simulink model "OfflineEstimator"  (R2020a)
settings: Solver=ode1be  StartTime=0.0  StopTime=simParams.duration.Value  FixedStep=0.00005  MaxStep=0.0005*sqrt(simParams.lengthScaleFactor.Value)  RelTol=1e-3  AbsTol=1e-3
undefined symbols (not defined in the file or in its folder): bridlePosVec, CMposVec, env, experimentalDataIsInput, externalDataIsInput, initPosKite, initVelKite, las, LEposIMU, linThrNodeCorrVec, NNodeTether, NNodeTether_cl, numObsThrNodes, obsLASphidotInit, obsLASphiInit, obsLASthetadotInit, obsLASthetaInit, ObsLink1DFlowVec, OBSTETHER, Obsthr, tow_start_time
libraries: vrlib x5, lineAngleSensor x5, dspsrcs4 x4, sharedutil x3, nodeDragForce_ul x3, nodeNetBuoyForce_ul x3, nodePosToLinkPos_ul x3, nodeSpringDamperForce_ul x3, eeGeneralControl x3, stateEstimation x3, dspsigops x3, thrNodeMass_ul x2
(part 1 of 2)
settings Model: SimulationMode=accelerator  PauseTimes=15  PacingRate=1000  ExtModeTrigDuration=100  Creator=mcobb  LastModifiedBy=Zak
settings SolverCC: AlgebraicLoopSolver=LineSearch  SolverResetMethod=Robust
settings DataIOCC: SaveFormat=StructureWithTime  SaveOutput=off  DSMLogging=off  StateSaveName=tmp_raccel_xout
settings OptimizationCC: EfficientMapNaN2IntZero=off
settings DebuggingCC: SignalRangeChecking=error  AlgebraicLoopMsg=none  ArtificialAlgebraicLoopMsg=none  ArithmeticOperatorsInVariantConditions=warning
settings HardwareCC: TargetBitPerPointer=64  TargetBitPerSizeT=64  TargetBitPerPtrDiffT=64  TargetLongLongMode=on  TargetIntDivRoundTo=Zero  TargetEndianess=LittleEndian  TargetWordSize=64  TargetHWDeviceType=MATLAB Host  ProdEqTarget=off
settings SFSimCC: CustomCodeUndefinedFunction=UseInterfaceOnly
settings CodeAppCC: MaxIdLength=128
settings GRTTargetCC: CombineOutputUpdateFcns=off  GRTInterface=on

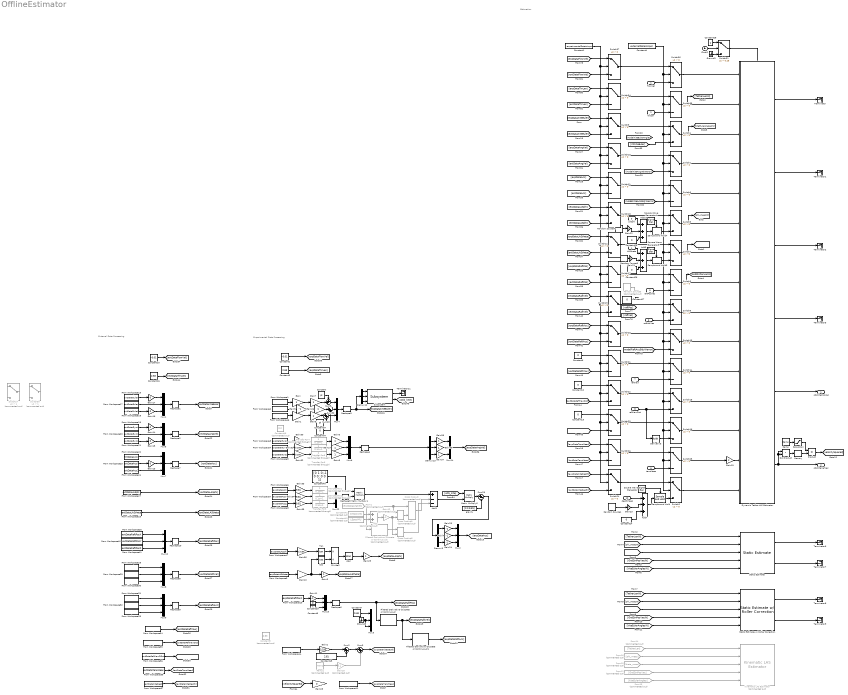
== system OfflineEstimator ==
  note: Estimation
  note: Experimental Data Processing
  note: External Data Processing
  flowVel : Inport
  thrLen : Inport  Port=2
  LASphi : Inport  Port=3
  LAStheta : Inport  Port=4
  raftPosVec : Inport  Port=5
  raftVelVec : Inport  Port=6
  raftYaw : Inport  Port=7
  raftYawDot : Inport  Port=8
  tensMeas : Inport  Port=9
  depthMeas : Inport  Port=10
  Add : Sum  Commented=on
  Add1 : Sum  Inputs=+--
  Add10 : Sum  Inputs=+++
  Add7 : Sum  Inputs=+++
  Add9 : Sum  Inputs=+++
  Atan : Trigonometry  Operator=atan
  Clock2 : Clock
  Constant : Constant  Value=pi
  Constant1 : Constant  Value=experimentalDataIsInput
  Constant10 : Constant  Value=-0.01
  Constant{6,12..13,24..27,29,47} (9 alike) : Constant  Value=0
  Constant16 : Constant  Value=2.63
  Constant2 : Constant  Value=-0.01
  Constant28 : Constant
  Constant3 : Constant  Value=2.63
  Constant37 : Constant  Value=pi
  Constant4 : Constant  Value=externalDataIsInput
  Constant40 : Constant  Value=[0 1 0;-1 0 0; 0 0 1]
  Constant42 : Constant  Commented=on  Value=CMposVec
  Constant43 : Constant  Commented=on  Value=LEposIMU
  Constant45 : Constant  Value=2.81
  Constant46 : Constant  Commented=on  Value=0.2
  Constant5 : Constant  Commented=on  Value=2.63
  Constant7 : Constant  Value=0.48
  Constant8 : Constant  Value=3
  Cos : Trigonometry  Operator=cos
  Cross Product : vrlib/Utilities/Cross Product  Commented=on
  Cross Product1 : vrlib/Utilities/Cross Product  Commented=on
  Cross Product2 : vrlib/Utilities/Cross Product  Commented=on
  Demux12 : Demux  Outputs=3
  Demux13 : Demux  Outputs=3
  Demux3 : Demux  Outputs=3
  Derivative : Derivative
  Divide2 : Product  Inputs=*/
  Dot Product : DotProduct  InputSameDT=on  OutDataTypeStr=Inherit: Inherit via internal rule
  Dynamic Tether LAS Estimator : Subsystem  AncestorBlock=lineAngleSensorObserver/lineAngleSensorObserver  mask{las=las, env=env}
      mask prompts: las "LAS Object"; env "Environment"
  Filtered Derivative (Discrete or Continuous) : eeGeneralControl/Filtered Derivative (Discrete or Continuous)  K=1  T=0.5  B=inf  A=-inf  minRatio=10  init_option=Inherited from block input  x0=0  Ts=-1
      settings: SourceProductBaseCode=PS
  Filtered Derivative (Discrete or Continuous)1 : eeGeneralControl/Filtered Derivative (Discrete or Continuous)  K=1  T=0.5  B=inf  A=-inf  minRatio=10  init_option=Inherited from block input  x0=0  Ts=-1
      settings: SourceProductBaseCode=PS
  Filtered Derivative (Discrete or Continuous)2 : eeGeneralControl/Filtered Derivative (Discrete or Continuous)  Commented=on  K=1  T=0.5  B=inf  A=-inf  minRatio=10  init_option=Inherited from block input  x0=0  Ts=-1
      settings: SourceProductBaseCode=PS
  From Workspace1 : FromWorkspace  VariableName=expDataEulerX  SampleTime=0.001  Interpolate=off  ZeroCross=off  OutputAfterFinalValue=Holding final value
  From Workspace10 : FromWorkspace  VariableName=expDataRaftPosX  SampleTime=0.001  Interpolate=off  ZeroCross=off  OutputAfterFinalValue=Holding final value
  From Workspace11 : FromWorkspace  VariableName=expDataTensMeas  SampleTime=0.001  Interpolate=off  ZeroCross=off  OutputAfterFinalValue=Holding final value
  From Workspace14 : FromWorkspace  VariableName=expDataKiteDepth  SampleTime=0.001  Interpolate=off  ZeroCross=off  OutputAfterFinalValue=Holding final value
  From Workspace15 : FromWorkspace  VariableName=extDataEulerX  SampleTime=0.001  Interpolate=off  ZeroCross=off  OutputAfterFinalValue=Holding final value
  From Workspace17 : FromWorkspace  VariableName=extDataEulerY  SampleTime=0.001  Interpolate=off  ZeroCross=off  OutputAfterFinalValue=Holding final value
  From Workspace18 : FromWorkspace  VariableName=extDataEulerZ  SampleTime=0.001  Interpolate=off  ZeroCross=off  OutputAfterFinalValue=Holding final value
  From Workspace19 : FromWorkspace  VariableName=extDataGyroX  SampleTime=0.001  Interpolate=off  ZeroCross=off  OutputAfterFinalValue=Holding final value
  From Workspace2 : FromWorkspace  VariableName=expDataEulerY  SampleTime=0.001  Interpolate=off  ZeroCross=off  OutputAfterFinalValue=Holding final value
  From Workspace20 : FromWorkspace  VariableName=extDataGyroY  SampleTime=0.001  Interpolate=off  ZeroCross=off  OutputAfterFinalValue=Holding final value
  From Workspace21 : FromWorkspace  VariableName=extDataGyroZ  SampleTime=0.001  Interpolate=off  ZeroCross=off  OutputAfterFinalValue=Holding final value
  From Workspace22 : FromWorkspace  VariableName=extDataAccX  SampleTime=0.001  Interpolate=off  ZeroCross=off  OutputAfterFinalValue=Holding final value
  From Workspace23 : FromWorkspace  VariableName=extDataAccY  SampleTime=0.001  Interpolate=off  ZeroCross=off  OutputAfterFinalValue=Holding final value
  From Workspace24 : FromWorkspace  VariableName=extDataAccZ  SampleTime=0.001  Interpolate=off  ZeroCross=off  OutputAfterFinalValue=Holding final value
  From Workspace25 : FromWorkspace  VariableName=extDataLAStheta  SampleTime=0.001  Interpolate=off  ZeroCross=off  OutputAfterFinalValue=Holding final value
  From Workspace26 : FromWorkspace  VariableName=extDataRaftPosX  SampleTime=0.001  Interpolate=off  ZeroCross=off  OutputAfterFinalValue=Holding final value
  From Workspace27 : FromWorkspace  VariableName=extDataLASphi  SampleTime=0.001  Interpolate=off  ZeroCross=off  OutputAfterFinalValue=Holding final value
  From Workspace28 : FromWorkspace  VariableName=extDataRaftVelX  SampleTime=0.001  Interpolate=off  ZeroCross=off  OutputAfterFinalValue=Holding final value
  From Workspace29 : FromWorkspace  VariableName=extDataRaftVelY  SampleTime=0.001  Interpolate=off  ZeroCross=off  OutputAfterFinalValue=Holding final value
  From Workspace3 : FromWorkspace  VariableName=expDataGyroX  SampleTime=0.001  Interpolate=off  ZeroCross=off  OutputAfterFinalValue=Holding final value
  From Workspace30 : FromWorkspace  VariableName=extDataRaftVelZ  SampleTime=0.001  Interpolate=off  ZeroCross=off  OutputAfterFinalValue=Holding final value
  From Workspace31 : FromWorkspace  VariableName=extDataRaftAccX  SampleTime=0.001  Interpolate=off  ZeroCross=off  OutputAfterFinalValue=Holding final value
  From Workspace32 : FromWorkspace  VariableName=extDataRaftAccY  SampleTime=0.001  Interpolate=off  ZeroCross=off  OutputAfterFinalValue=Holding final value
  From Workspace33 : FromWorkspace  VariableName=extDataRaftAccZ  SampleTime=0.001  Interpolate=off  ZeroCross=off  OutputAfterFinalValue=Holding final value
  From Workspace34 : FromWorkspace  VariableName=extDataRaftYaw  SampleTime=0.001  Interpolate=off  ZeroCross=off  OutputAfterFinalValue=Holding final value
  From Workspace35 : FromWorkspace  VariableName=extDataRaftYawDot  SampleTime=0.001  Interpolate=off  ZeroCross=off  OutputAfterFinalValue=Holding final value
  From Workspace36 : FromWorkspace  VariableName=extDataRaftYawDDot  SampleTime=0.001  Interpolate=off  ZeroCross=off  OutputAfterFinalValue=Holding final value
  From Workspace37 : FromWorkspace  VariableName=extDataKiteDepth  SampleTime=0.001  Interpolate=off  ZeroCross=off  OutputAfterFinalValue=Holding final value
  From Workspace39 : FromWorkspace  VariableName=extDataTensMeas  SampleTime=0.001  Interpolate=off  ZeroCross=off  OutputAfterFinalValue=Holding final value
  From Workspace4 : FromWorkspace  VariableName=expDataGyroY  SampleTime=0.001  Interpolate=off  ZeroCross=off  OutputAfterFinalValue=Holding final value
  From Workspace40 : FromWorkspace  VariableName=extDataRaftPosY  SampleTime=0.001  Interpolate=off  ZeroCross=off  OutputAfterFinalValue=Holding final value
  From Workspace41 : FromWorkspace  VariableName=extDataRaftPosZ  SampleTime=0.001  Interpolate=off  ZeroCross=off  OutputAfterFinalValue=Holding final value
  From Workspace46 : FromWorkspace  VariableName=expDataEulerZ  SampleTime=0.001  Interpolate=off  ZeroCross=off  OutputAfterFinalValue=Holding final value
  From Workspace47 : FromWorkspace  VariableName=expDataLASphi  SampleTime=0.001  Interpolate=off  ZeroCross=off  OutputAfterFinalValue=Holding final value
  From Workspace5 : FromWorkspace  VariableName=expDataGyroZ  SampleTime=0.001  Interpolate=off  ZeroCross=off  OutputAfterFinalValue=Holding final value
  From Workspace6 : FromWorkspace  VariableName=expDataAccX  SampleTime=0.001  Interpolate=off  ZeroCross=off  OutputAfterFinalValue=Holding final value
  From Workspace7 : FromWorkspace  VariableName=expDataAccY  SampleTime=0.001  Interpolate=off  ZeroCross=off  OutputAfterFinalValue=Holding final value
  From Workspace8 : FromWorkspace  VariableName=expDataAccZ  SampleTime=0.001  Interpolate=off  ZeroCross=off  OutputAfterFinalValue=Holding final value
  From Workspace9 : FromWorkspace  VariableName=expDataLAStheta  SampleTime=0.001  Interpolate=off  ZeroCross=off  OutputAfterFinalValue=Holding final value
  From1 : From  Commented=on  GotoTag=expDataAngVel
  From12 : From  Commented=on  GotoTag=GndStnPosVec
  From13 : From  Commented=on  GotoTag=kiteEulerAngles
  From14 : From  Commented=on  GotoTag=TetherLen
  From15 : From  Commented=on  GotoTag=theta_meas
  From16 : From  Commented=on  GotoTag=phi_meas
  Gain{,3,5..8,26..27,29,37..39} (12 alike) : Gain
  Gain1 : Gain  Gain=-pi/180
  Gain10 : Gain  Gain=-pi/180
  Gain{4,9,11,24..25} (5 alike) : Gain  Gain=-1
  Gain12 : Gain  Commented=on  Gain=-1
  Gain{13..17,21..23,28} (9 alike) : Gain  Gain=0
  Gain18 : Gain  Commented=on  Gain=0.1
  Gain19 : Gain  Gain=2
  Gain2 : Gain  Gain=-1/100
  Gain{30..32,36} (4 alike) : Gain  Gain=pi/180
  Gain33 : Gain  Gain=9.81
  Gain34 : Gain  Gain=9.81
  Gain35 : Gain  Gain=9.81
  Ground3 : Ground
  Ground8 : Ground
  Kinematic LAS Estimator : stateEstimation/State Estimation/Kinematic LAS Estimator  Commented=on  SystemSampleTime=-1  Latency=0  AutoFrameSizeCalculation=off
  Matrix Multiply1 : Product  Multiplication=Matrix(*)
  Matrix Multiply6 : Product  Multiplication=Matrix(*)
  Memory : Memory
  Mux{1..10,22..24} (13 alike) : Mux  Inputs=3
  Product : Product
  Ramp : simulink/Sources/Ramp  slope=0.1  start=0  InitialOutput=0
  Ramp1 : simulink/Sources/Ramp  Commented=on  slope=0.5  start=10  InitialOutput=0
  Random Source1 : dspsrcs4/Random Source  SrcType=Gaussian  NormMethod=Ziggurat  CltLength=12  MinVal=0  MaxVal=1  MeanVal=0  VarVal=1e-6  RepMode=Not repeatable  rawSeed=1  IsInherit=off  SampMode=Continuous  SampTime=0.01  SampFrame=1  DataType=Double  OutComplex=Real  OutputFrames=off
  Random Source3 : dspsrcs4/Random Source  SrcType=Gaussian  NormMethod=Ziggurat  CltLength=12  MinVal=0  MaxVal=1  MeanVal=0  VarVal=(0.01*3.14/180)^2  RepMode=Not repeatable  rawSeed=1  IsInherit=off  SampMode=Continuous  SampTime=0.01  SampFrame=1  DataType=Double  OutComplex=Real  OutputFrames=off
  Random Source4 : dspsrcs4/Random Source  SrcType=Gaussian  NormMethod=Ziggurat  CltLength=12  MinVal=0  MaxVal=1  MeanVal=0  VarVal=(0.01*3.14/180)^2  RepMode=Not repeatable  rawSeed=1  IsInherit=off  SampMode=Continuous  SampTime=0.01  SampFrame=1  DataType=Double  OutComplex=Real  OutputFrames=off
  Random Source5 : dspsrcs4/Random Source  Commented=on  SrcType=Gaussian  NormMethod=Ziggurat  CltLength=12  MinVal=0  MaxVal=1  MeanVal=0  VarVal=1e-6  RepMode=Not repeatable  rawSeed=1  IsInherit=off  SampMode=Continuous  SampTime=0.01  SampFrame=1  DataType=Double  OutComplex=Real  OutputFrames=off
  Reshape{1..10} (10 alike) : Reshape  OutputDimensionality=Column vector (2-D)
  Sample and Hold : dspsigops/Sample and Hold  trig=Rising edge  initCond=0  latchinput=off
  Sample and Hold3 : dspsigops/Sample and Hold  trig=Rising edge  initCond=0  latchinput=off
  Sample and Hold4 : dspsigops/Sample and Hold  trig=Rising edge  initCond=0  latchinput=off
  Saturation : Saturate  UpperLimit=1  LowerLimit=0
  Square Wave Generator : SignalGenerator  WaveForm=square  Frequency=25
  Square Wave Generator3 : SignalGenerator  WaveForm=square  Frequency=25
  Square Wave Generator4 : SignalGenerator  WaveForm=square  Frequency=25
  Static Estimate : stateEstimation/State Estimation/Static Estimate  SystemSampleTime=-1  Latency=0  AutoFrameSizeCalculation=off
  Static Estimate w/ Roller Correction : stateEstimation/State Estimation/Static Estimate w// Roller Correction  SystemSampleTime=-1  Latency=0  AutoFrameSizeCalculation=off
  Subsystem : lineAngleSensorObserver/lineAngleSensorObserver/Subsystem  SystemSampleTime=-1  Latency=0  AutoFrameSizeCalculation=off
  Sum{2..3,28,30} (4 alike) : Sum  Inputs=|++
  Sum29 : Sum  Inputs=|+-
  Sum5 : Sum  Inputs=++|
  Switch{1..26,34..37} (30 alike) : Switch  Criteria=u2 > Threshold
  Switch27 : Switch  Commented=on  Criteria=u2 > Threshold  Threshold=1
  Switch30 : Switch  Commented=on  Criteria=u2 > Threshold  Threshold=1
  Switch31 : Switch  Criteria=u2 > Threshold  Threshold=0.25
  Tan : Trigonometry  Operator=tan
  Terminator{,1..3,6..9,11} (9 alike) : Terminator
  Transfer Fcn{1..6} (6 alike) : TransferFcn  Commented=through  Denominator=[0.1 1]
  gravity : Constant  Value=[0 0 9.81]
  obsKitePosVec : Outport
  obsKiteVelVec : Outport  Port=2
  wires:
  raftYaw/1 -> Switch14/3
  Switch3/1 -> [GndStnPosVecIN], Dynamic Tether LAS Estimator/8(raftPos)  "obsIN_RaftPos"
  Switch35/1 -> Dynamic Tether LAS Estimator/2(thrLen), [TetherLenIN]  "obsIN_obsThrLen"
  Constant4/1 -> Switch36/2, Switch35/2, Switch1/2, Switch6/2, Switch5/2, Switch7/2, Switch3/2, Switch13/2, Switch14/2, Switch15/2, Switch25/2, Switch2/2, Switch16/2, Switch8/2, Switch4/2
  Dynamic Tether LAS Estimator/2(phiDot) -> Terminator1/1  "obsOUT_LASphiDot"
  Dynamic Tether LAS Estimator/5(estKitePos) -> obsKitePosVec/1  "obsOUT_kitePosVec"
  Derivative/1 -> Switch16/3
  [extDataRaftYaw] -> Switch21/3
  Switch6/1 -> Dynamic Tether LAS Estimator/5(KiteAcc)  "obsIN_kiteAcc"
  Switch26/1 -> Switch25/1
  From Workspace41/1 -> Mux10/3
  From Workspace34/1 -> [extDataRaftYaw]
  Switch1/1 -> Dynamic Tether LAS Estimator/4(kiteAngVel)  "obsIN_kiteAngVel"
  Switch21/1 -> Switch14/1
  Constant6/1 -> Switch21/1
  Static Estimate w/ Roller Correction/1 -> Terminator8/1  "staticEstRollerOut_kitePosVec"
  Switch19/1 -> Switch8/1
  From Workspace29/1 -> Mux8/2
  From Workspace18/1 -> Gain16/1
  From Workspace17/1 -> Mux1/2
  Reshape10/1 -> [extDataRaftPos]
  Mux7/1 -> Reshape7/1
  Switch24/1 -> Switch2/1
  Mux5/1 -> Reshape2/1
  [expDataKiteEuler] -> Switch9/1
  From13/1 -> Kinematic LAS Estimator/5
  From16/1 -> Kinematic LAS Estimator/2
  Static Estimate w/ Roller Correction/2 -> Terminator9/1  "staticEstRollerOut_kiteVelVec"
  From12/1 -> Kinematic LAS Estimator/4
  From Workspace37/1 -> [extDataKiteDepth]
  [kiteEulerAnglesIN] -> Static Estimate w/ Roller Correction/5
  [kiteEulerAnglesIN] -> Static Estimate/5  "staticEstIn_eulerAnglesKite"
  From Workspace25/1 -> [extDataLAStheta]
  [theta_measIN] -> Static Estimate w/ Roller Correction/3
  flowVel/1 -> Switch36/3  "obsIN_flowVel"
  Switch4/1 -> Dynamic Tether LAS Estimator/3(kiteEulerAngles), [kiteEulerAnglesIN]  "obsIN_KiteEulerAngles"
  From Workspace21/1 -> Gain15/1
  Switch37/1 -> Switch36/1
  [extDataFlowVel] -> Switch37/3
  Gain22/1 -> Add10/2
  From Workspace15/1 -> Gain17/1
  Gain23/1 -> Add7/2
  [expDataAcc] -> Switch11/1
  From Workspace33/1 -> Mux9/3
  From Workspace26/1 -> Mux10/1
  Switch2/1 -> Dynamic Tether LAS Estimator/15(depthMeas)  "obsIN_kiteDepth"
  Switch9/1 -> Switch4/1
  Constant12/1 -> Switch22/1
  [extDataKiteDepth] -> Switch24/3
  Switch8/1 -> Dynamic Tether LAS Estimator/9(raftVel)  "obsIN_RaftVel"
  From Workspace28/1 -> Mux8/1
  [expDataRaftVel] -> Switch19/1
  tensMeas/1 -> Switch25/3
  From Workspace40/1 -> Mux10/2
  Switch13/1 -> Dynamic Tether LAS Estimator/10(raftAcc)  "obsIN_RaftAcc"
  From14/1 -> Kinematic LAS Estimator/1
  Square Wave Generator4/1 -> Sample and Hold4/Trigger
  Switch23/1 -> Switch16/1
  From Workspace23/1 -> Gain13/1
  [expDataTensMeas] -> Switch26/1
  Clock2/1 -> Switch31/2
  [modelKiteAccBdyWerror] -> Switch6/3
  Sample and Hold4/1 -> Switch5/3
  LASphi/1 -> Add10/1
  Mux10/1 -> Reshape10/1
  Switch36/1 -> Dynamic Tether LAS Estimator/1(flowSpd)  "obsIN_flowVel"
  Add10/1 -> Sample and Hold4/1
  Mux8/1 -> Reshape8/1
  Sample and Hold/1 -> Switch2/3
  Sample and Hold3/1 -> Switch7/3
  Static Estimate/2 -> Terminator7/1  "staticEstOut_kiteVelVec"
  From Workspace19/1 -> Gain14/1
  Constant28/1 -> Switch31/1
  Switch18/1 -> Switch5/1
  Random Source4/1 -> Gain22/1
  Random Source3/1 -> Gain21/1
  Constant26/1 -> Add9/3
  From Workspace31/1 -> Mux9/1
  Ground3/1 -> Switch31/3
  Switch10/1 -> Switch1/1
  Constant25/1 -> Add10/3
  Switch17/1 -> Switch3/1
  Square Wave Generator/1 -> Sample and Hold/Trigger
  Dynamic Tether LAS Estimator/1(phi) -> Terminator/1  "obsOUT_LASphi"
  Reshape7/1 -> [extDataAcc]
  [extDataRaftYawDot] -> Switch22/3
  From15/1 -> Kinematic LAS Estimator/3
  [expDataThrLen] -> Switch34/1
  depthMeas/1 -> Add7/1
  Dynamic Tether LAS Estimator/3(theta) -> Terminator2/1  "obsOUT_LAStheta"
  From Workspace36/1 -> [extDataRaftYawDDot]
  Switch12/1 -> Switch7/1
  [phi_measIN] -> Static Estimate w/ Roller Correction/2
  [expDataLASphi] -> Switch18/1
  Switch14/1 -> Dynamic Tether LAS Estimator/11(raftPsi)  "obsIN_RaftYaw"
  Random Source1/1 -> Gain23/1
  From Workspace27/1 -> [extDataLASphi]
  [extDataTensMeas] -> Switch26/3
  Static Estimate/1 -> Terminator6/1  "staticEstOut_kitePosVec"
  Dynamic Tether LAS Estimator/6(estKiteVel) -> obsKiteVelVec/1, Dot Product/1, Dot Product/2  "obsOUT_kiteVelVec"
  [extDataThrLen] -> Switch34/3
  Switch20/1 -> Switch13/1
  Dynamic Tether LAS Estimator/4(thetaDot) -> Terminator3/1  "obsOUT_LASthetaDot"
  Switch16/1 -> Dynamic Tether LAS Estimator/13(raftPsiDDot)  "obsIN_RaftYawDDot"
  Reshape8/1 -> [extDataRaftVel]
  Reshape1/1 -> [extDataKiteEuler]
  From Workspace24/1 -> Mux7/3
  From Workspace20/1 -> Mux5/2
  Switch7/1 -> [theta_measIN], Dynamic Tether LAS Estimator/7(LASthetaMeas)  "obsIN_LASthetaMeas"
  From Workspace22/1 -> Mux7/1
  [extDataRaftAcc] -> Switch20/3
  Switch15/1 -> Dynamic Tether LAS Estimator/12(raftPsiDot)  "obsIN_RaftYawDot"
  Constant13/1 -> Switch23/1
  [GndStnPosVecIN] -> Static Estimate/4  "staticEstIn_raftPosVec"
  [expDataLAStheta] -> Switch12/1
  Constant10/1 -> [extDataFlowVel]
  Add7/1 -> Sample and Hold/1
  Add9/1 -> Sample and Hold3/1
  [extDataRaftVel] -> Switch19/3
  From Workspace35/1 -> [extDataRaftYawDot]
  [extDataKiteEuler] -> Switch9/3
  raftVelVec/1 -> Switch8/3
  [TetherLenIN] -> Static Estimate/1  "staticEstIn_thrLen"
  LAStheta/1 -> Add9/1
  [extDataRaftPos] -> Switch17/3
  [extDataLASphi] -> Switch18/3
  [expDataAngVel] -> Switch10/1
  [expDataFlowVel] -> Switch37/1
  Reshape9/1 -> [extDataRaftAcc]
  [phi_measIN] -> Static Estimate/2  "staticEstIn_phiLAS"
  [extDataLAStheta] -> Switch12/3
  [expDataRaftAcc] -> Switch20/1
  Reshape2/1 -> [extDataAngVel]
  Gain21/1 -> Add9/2
  Mux9/1 -> Reshape9/1
  Constant24/1 -> Add7/3
  [theta_measIN] -> Static Estimate/3  "staticEstIn_thetaLAS"
  [extDataAcc] -> Switch11/3
  Switch5/1 -> Dynamic Tether LAS Estimator/6(LASphiMeas), [phi_measIN]  "obsIN_LASphiMeas"
  Square Wave Generator3/1 -> Sample and Hold3/Trigger
  Constant27/1 -> ?
  Switch31/1 -> ?
  Random Source5/1 -> ?
  From Workspace30/1 -> Mux8/3
  [CFkiteEuler] -> Switch4/3
  From Workspace32/1 -> Mux9/2
  Constant1/1 -> Switch37/2, Switch34/2, Switch26/2, Switch24/2, Switch23/2, Switch22/2, Switch21/2, Switch20/2, Switch19/2, Switch17/2, Switch12/2, Switch18/2, Switch11/2, Switch10/2, Switch9/2
  raftPosVec/1 -> Switch3/3
  [expDataRaftPos] -> Switch17/1
  raftYawDot/1 -> Switch15/3, Derivative/1
  thrLen/1 -> Switch35/3  "obsIN_obsThrLen"
  Constant16/1 -> [extDataThrLen]
  [GndStnPosVecIN] -> Static Estimate w/ Roller Correction/4
  From Workspace39/1 -> [extDataTensMeas]
  [modelKiteAngVelWerror] -> Switch1/3
  [modelRaftAccBdyWerror] -> Switch13/3
  [TetherLenIN] -> Static Estimate w/ Roller Correction/1
  Switch22/1 -> Switch15/1
  Switch34/1 -> Switch35/1
  [extDataRaftYawDDot] -> Switch23/3
  Switch11/1 -> Switch6/1
  Switch25/1 -> Gain19/1  "obsIN_tensMeas"
  [extDataAngVel] -> Switch10/3
  Mux1/1 -> Reshape1/1
  [expDataKiteDepth] -> Switch24/1
  Dot Product/1 -> Memory/1
  Memory/1 -> Product/2
  Product/1 -> [velocitySquared]
  Ramp/1 -> Saturation/1
  Saturation/1 -> Product/1
  Filtered Derivative (Discrete or Continuous)2/1 -> Cross Product2/1
  Mux2/1 -> [expDataAcc]
  Cross Product2/1 -> Add1/3
  Gain9/1 -> Gain26/1
  Sum28/1 -> Mux4/3
  Constant42/1 -> Add/1
  Gain24/1 -> Mux2/3
  From Workspace5/1 -> Gain32/1
  From Workspace1/1 -> Gain/1
  Gain35/1 -> Transfer Fcn3/1
  Mux4/1 -> Reshape3/1
  From Workspace14/1 -> Gain2/1  "depth_cm"
  From Workspace10/1 -> Gain11/1
  Cross Product1/1 -> Cross Product/2
  Add1/1 -> Matrix Multiply6/2
  Cos/1 -> Divide2/2
  Gain10/1 -> Gain3/1, Cos/1
  From Workspace6/1 -> Gain33/1
  [oCb_kite] -> Matrix Multiply6/1
  Gain32/1 -> Transfer Fcn6/1
  Gain33/1 -> Transfer Fcn1/1
  Constant8/1 -> Mux23/3
  From Workspace3/1 -> Gain30/1
  Cross Product/1 -> Add1/2
  Demux3/1 -> Gain25/1
  Gain2/1 -> Sum2/1  "depth_m"
  Sum2/1 -> Sum3/1
  Demux3/2 -> Gain4/1
  Gain3/1 -> [expDataLAStheta]
  Gain26/1 -> Sum30/1
  Atan/1 -> Gain29/1
  From Workspace47/1 -> Gain36/1
  Constant/1 -> Sum5/1
  Tan/1 -> Divide2/1
  Transfer Fcn6/1 -> Gain8/1
  Gain36/1 -> Tan/1
  Gain/1 -> Gain7/1
  Transfer Fcn4/1 -> Gain6/1
  From Workspace7/1 -> Gain34/1
  Subsystem/1 -> Terminator11/1
  From1/1 -> Filtered Derivative (Discrete or Continuous)2/1, Cross Product/1, Cross Product1/1
  Sum29/1 -> Demux3/1
  Gain5/1 -> Sum28/1
  Ground8/1 -> Mux3/3, Mux3/2
  Gain25/1 -> Mux2/1
  Filtered Derivative (Discrete or Continuous)1/1 -> [expDataRaftAcc]
  Divide2/1 -> Atan/1
  Gain31/1 -> Transfer Fcn5/1
  Constant29/1 -> Mux23/2
  Transfer Fcn3/1 -> Mux22/3
  Gain12/1 -> Cross Product2/2, Cross Product1/2
  From Workspace8/1 -> Gain35/1
  Gain7/1 -> Sum5/2
  Demux12/2 -> Subsystem/2
  Reshape6/1 -> [expDataRaftPos], Filtered Derivative (Discrete or Continuous)/1
  Subsystem/2 -> [oCb_kite]
  Gain11/1 -> Mux23/1
  Demux3/3 -> Gain24/1
  Transfer Fcn5/1 -> Gain27/1
  gravity/1 -> Sum29/2
  Gain29/1 -> [expDataLASphi]
  Constant47/1 -> Sum30/2
  Transfer Fcn2/1 -> Mux22/2
  Constant43/1 -> Add/2
  Matrix Multiply6/1 -> Sum29/1
  Reshape4/1 -> Demux13/1
  Sum30/1 -> Mux4/2
  Reshape5/1 -> Matrix Multiply1/2
  Gain39/1 -> Mux24/2
  Demux12/1 -> Subsystem/1
  Gain34/1 -> Transfer Fcn2/1
  Mux24/1 -> [expDataAngVel]
  Gain4/1 -> Mux2/2
  Demux12/3 -> Subsystem/3
  Demux13/3 -> Gain37/1
  Gain8/1 -> Mux6/3
  Filtered Derivative (Discrete or Continuous)/1 -> [expDataRaftVel], Filtered Derivative (Discrete or Continuous)1/1
  Constant40/1 -> Matrix Multiply1/1  "bCimu"
  Sum5/1 -> Mux4/1
  Gain6/1 -> Mux6/1
  Gain1/1 -> Gain5/1
  Demux13/2 -> Gain39/1
  Gain30/1 -> Transfer Fcn4/1
  Sum3/1 -> [expDataKiteDepth]
  Constant7/1 -> Mux3/1
  Demux13/1 -> Gain38/1
  Gain37/1 -> Mux24/3
  Constant3/1 -> [expDataThrLen]
  Reshape3/1 -> [expDataKiteEuler], Demux12/1
  Constant37/1 -> Sum28/2
  Constant45/1 -> Sum2/2
  Mux23/1 -> Reshape6/1
  Gain27/1 -> Mux6/2
  Matrix Multiply1/1 -> Add1/1
  Transfer Fcn1/1 -> Mux22/1
  Add/1 -> Gain12/1
  Mux22/1 -> Reshape5/1
  From Workspace4/1 -> Gain31/1
  Gain38/1 -> Mux24/1
  Mux6/1 -> Reshape4/1
  From Workspace2/1 -> Gain9/1
  From Workspace46/1 -> Gain1/1
  Constant2/1 -> [expDataFlowVel]
  [velocitySquared] -> Gain28/1
  Gain13/1 -> Mux7/2
  Gain14/1 -> Mux5/1
  Gain15/1 -> Mux5/3
  Gain16/1 -> Mux1/3
  Gain17/1 -> Mux1/1
  From Workspace11/1 -> [expDataTensMeas]  "tens_N"
  Gain18/1 -> Sum3/2
  Ramp1/1 -> Gain18/1
  Gain19/1 -> Dynamic Tether LAS Estimator/14(tensionMeas)
  From Workspace9/1 -> Gain10/1

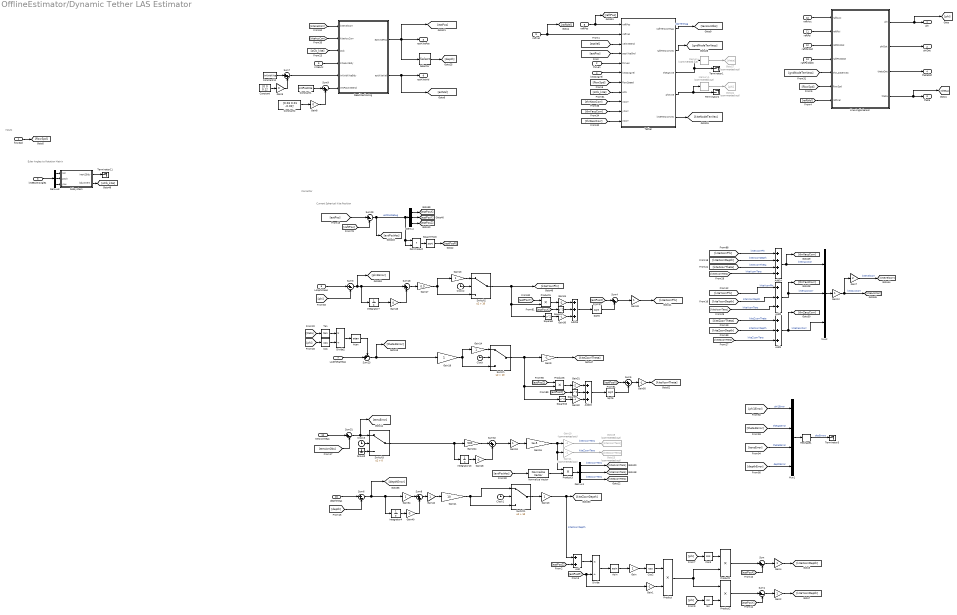
== system OfflineEstimator/Dynamic Tether LAS Estimator ==
  note: Corrector
  note: Current Spherical Kite Position
  note: Euler Angles to Rotation Matrix
  note: Inputs
  flowSpd : Inport
  thrLen : Inport  Port=2
  kiteEulerAngles : Inport  Port=3
  kiteAngVel : Inport  Port=4
  KiteAcc : Inport  Port=5
  LASphiMeas : Inport  Port=6
  LASthetaMeas : Inport  Port=7
  raftPos : Inport  Port=8
  raftVel : Inport  Port=9
  raftAcc : Inport  Port=10
  raftPsi : Inport  Port=11
  raftPsiDot : Inport  Port=12
  raftPsiDDot : Inport  Port=13
  tensionMeas : Inport  Port=14
  depthMeas : Inport  Port=15
  Add : Sum
  Add{1..2,13,15} (4 alike) : Sum  Inputs=3
  Add14 : Sum  Inputs=4
  Asin : Trigonometry  Operator=asin
  Atan : Trigonometry  Operator=atan
  Clock{,1..3} (4 alike) : Clock
  Constant : Constant  Value=[0 0 0.1]'
  Constant1 : Constant  Value=initPosKite
  Constant12 : Constant  Value=initVelKite
  Constant2 : Constant  Value=[0.03 0.01 -0.02]'
  Cos : Trigonometry  Operator=cos
  Cos2 : Trigonometry  Operator=cos
  Cos3 : Trigonometry  Operator=cos
  Dead Reckoning : Subsystem
  Demux : Demux  Outputs=3
  Demux1 : Demux  Outputs=3
  Demux3 : Demux  Outputs=3
  Divide : Product  Inputs=*/
  Divide2 : Product  Inputs=*/
  Dot Product : DotProduct  InputSameDT=on  OutDataTypeStr=Inherit: Inherit via internal rule
  Gain{,2,4,12..14,18..19,34,42..43,49} (12 alike) : Gain
  Gain{1,9,30,32,50} (5 alike) : Gain  Gain=-1
  Gain10 : Gain  Commented=on  Gain=-1
  Gain11 : Gain  Commented=on  Gain=-1
  Gain16 : Gain  Gain=1e-5
  Gain224 : Gain  Gain=500
  Gain24 : Gain  Gain=-2
  Gain31 : Gain  Gain=-2
  Gain{5,8,40,46,48} (5 alike) : Gain  Gain=0
  Gain41 : Gain  Gain=10
  Gain47 : Gain  Gain=0.5
  Gain7 : Gain  Gain=2
  Goto19 : Goto  Commented=on  GotoTag=kiteXcorrTens
  Goto23 : Goto  Commented=on  GotoTag=kiteZcorrTens
  Goto24 : Goto  Commented=on  GotoTag=phi
  Goto27 : Goto  Commented=on  GotoTag=theta
  Ground : Ground
  Integrator13 : Integrator
  Integrator4 : Integrator
  Integrator7 : Integrator
  Line Angle Sensor : Subsystem
  Memory : Memory  Commented=on
  Memory1 : Memory  Commented=on
  Mux1 : Mux
  Mux2 : Mux  Inputs=3
  Normalize Vector : vrlib/Utilities/Normalize Vector  maxzero=0
  Product{,1..3,5..6} (6 alike) : Product
  Reshape1 : Reshape  OutputDimensionality=Column vector (2-D)
  Selector : Selector  InputPortWidth=3  IndexOptions=Index vector (dialog)  Indices=[3]  OutputSizes=1
  Sin : Trigonometry
  Sqrt5 : Sqrt  SaturateOnIntegerOverflow=on
  Sqrt6 : Sqrt  SaturateOnIntegerOverflow=on
  Square Root : Sqrt  SaturateOnIntegerOverflow=on
  Square{7..10} (4 alike) : Math  Operator=square  SaturateOnIntegerOverflow=on
  Subsystem : Subsystem
  Sum{,1,3,6,29,31} (6 alike) : Sum  Inputs=|+-
  Sum{4..5,7..9,18,32} (7 alike) : Sum  Inputs=|++
  Sum23 : Sum  Inputs=-+|
  Switch : Switch  Criteria=u2 > Threshold  Threshold=10
  Switch1 : Switch  Criteria=u2 > Threshold  Threshold=10
  Switch2 : Switch  Criteria=u2 > Threshold  Threshold=10
  Switch3 : Switch  Criteria=u2 > Threshold
  Tan : Trigonometry  Operator=tan
  Terminator{1..3,11} (4 alike) : Terminator
  Tether : Subsystem
  phi : Outport
  phiDot : Outport  Port=2
  theta : Outport  Port=3
  thetaDot : Outport  Port=4
  estKitePos : Outport  Port=5
  estKiteVel : Outport  Port=6
  wires:
  Gain8/1 -> Sum9/2
  Gain5/1 -> Sum7/2
  Constant2/1 -> Gain8/1
  Sum9/1 -> Dead Reckoning/6(initPosKiteGnd)
  Sum7/1 -> Dead Reckoning/5(initVelKiteBdy)
  Constant/1 -> Gain5/1
  Tether/3(thetaKine) -> Memory/1, Terminator1/1
  Tether/4(phiKine) -> Memory1/1, Terminator2/1
  Gain4/1 -> [kiteXcorrDepth]
  Gain2/1 -> [kiteYcorrDepth]
  [kiteYcorrDepth] -> Add2/2  "kiteYcorrDepth"
  Add2/1 -> Mux2/2, [thrYaccCorr]  "kiteYaccCorr"
  Sum1/1 -> Gain2/1
  Sum/1 -> Gain4/1
  [estPosY] -> Sum1/2
  [estPosX] -> Sum/2
  Product2/1 -> Sum1/1
  Product1/1 -> Sum/1
  [phi] -> Sin/1
  [phi] -> Cos3/1
  Sin/1 -> Product2/2
  Cos3/1 -> Product1/1
  Product/1 -> Product1/2, Product2/1
  Gain1/1 -> Product/2
  Cos2/1 -> Product/1
  Gain/1 -> Cos2/1
  Asin/1 -> Gain/1
  Divide/1 -> Asin/1
  [estPosR] -> Divide/2, Gain1/1
  Square Root/1 -> [estPosR]
  Dot Product/1 -> Square Root/1
  Add/1 -> Divide/1
  [estPosZ] -> Add/2
  [kiteVelCorr] -> Dead Reckoning/1(kiteVelCorr)
  Dead Reckoning/2(estKiteVel) -> estKiteVel/1, [estVel]
  Constant1/1 -> Sum9/1
  [kiteAccCorr] -> Dead Reckoning/2(kiteAccCorr)
  Dead Reckoning/1(estKitePos) -> estKitePos/1, [estPos], Selector/1
  KiteAcc/1 -> Dead Reckoning/4(KiteAccBdy)
  Constant12/1 -> Sum7/1
  [oCb_kite] -> Dead Reckoning/3(oCb)
  Selector/1 -> [depth]
  [flowSpd] -> Tether/7(flowSpeed)
  Tether/1(raftTensionMag) -> [tensionObs]  "obsTenMag"
  kiteAngVel/1 -> Tether/6(kiteAngVel)
  thrLen/1 -> Tether/5(thrLen)
  raftPos/1 -> [raftPos], Tether/1(raftPos)
  [oCb_kite] -> Tether/8(oCb)
  Tether/2(raftTensionVec) -> [gndNodeTenVecs]
  [estVel] -> Tether/3(velKiteGnd)
  [estPos] -> Tether/4(posKiteGnd)
  raftVel/1 -> [raftVel], Tether/2(raftVel)
  Add1/1 -> [thrZaccCorr], Mux2/3  "kiteZaccCorr"
  Sum8/1 -> Gain42/1
  Product5/1 -> Gain24/1
  Switch2/1 -> Product5/2, Square8/1, [kiteYcorrPhi]
  [kiteZcorrTheta] -> Add1/1  "kiteZcorrTheta"
  [kiteXcorrPhi] -> Add14/1  "kiteXcorrPhi"
  Demux/2 -> [estPosY]
  [estPosX] -> Sum5/1
  Gain50/1 -> [kiteXcorrTheta]
  [raftPos] -> Sum29/2
  Sum3/1 -> Integrator7/1, Sum18/1, [phi1Error]
  Demux/1 -> [estPosX]
  Reshape1/1 -> Terminator3/1  "obsErrors"
  Gain48/1 -> Sum32/2
  Demux/3 -> [estPosZ]
  depthMeas/1 -> Sum6/1
  [depth] -> Sum6/2
  Square8/1 -> Gain30/1
  Integrator13/1 -> Gain48/1
  [estPosX] -> Square7/1
  Gain24/1 -> Add13/1
  Square7/1 -> Add13/2
  Add14/1 -> [thrXaccCorr], Mux2/1  "kiteXaccCor"
  Gain31/1 -> Add15/1
  [kiteXcorrTheta] -> Add14/3  "kiteXcorrTheta"
  Sum29/1 -> [extPosVec], Demux/1, Dot Product/2, Dot Product/1  "estPosDebug"
  [kiteXcorrDepth] -> Add14/2  "kiteXcorrDepth"
  Gain12/1 -> [kiteAccCorr], Gain7/1  "kiteAccCorr"
  [kiteZcorrDepth] -> Add1/2  "kiteZcorrDepth"
  [estPosX] -> Square9/1
  Square10/1 -> Gain32/1
  Sum18/1 -> Gain47/1
  Gain32/1 -> Add15/3
  Sqrt6/1 -> Sum5/2
  Sqrt5/1 -> Sum4/2
  Sum4/1 -> Gain49/1
  Switch/1 -> Square10/1, Product6/2, Gain9/1
  Add13/1 -> Sqrt5/1
  [depthError] -> Mux1/4  "depthError"
  [estPosY] -> Product5/1
  [estPosZ] -> Product6/1
  Gain46/1 -> Sum18/2
  Add15/1 -> Sqrt6/1
  Product6/1 -> Gain31/1
  Sum23/1 -> Gain19/1, [theta1Error]
  Gain16/1 -> Gain10/1, Product3/1, Gain11/1
  [tensionObs] -> Sum31/2
  Switch3/1 -> Integrator13/1, Gain224/1
  Sum6/1 -> Integrator4/1, Gain34/1, [depthError]
  Gain7/1 -> [kiteVelCorr]  "kiteVelCorr"
  Gain42/1 -> Gain41/1
  Demux1/1 -> [kiteXcorrTens]  "kiteXcorrTens"
  Gain40/1 -> Sum8/2
  Integrator4/1 -> Gain40/1
  Gain224/1 -> Sum32/1
  [phi] -> Sum3/2
  Gain18/1 -> Gain16/1
  [kiteYcorrPhi] -> Add2/1  "kiteYcorrPhi"
  Gain30/1 -> Add13/3
  [tensError] -> Mux1/3  "theta2Error"
  Square9/1 -> Add15/2
  LASphiMeas/1 -> Sum3/1
  [phi1Error] -> Mux1/1  "phi1Error"
  Mux1/1 -> Reshape1/1
  [theta1Error] -> Mux1/2  "theta1Error"
  Integrator7/1 -> Gain46/1
  Demux1/3 -> [kiteZcorrTens]  "kiteZcorrTens"
  [estPos] -> Sum29/1
  Sum5/1 -> Gain50/1
  Gain43/1 -> [kiteZcorrDepth], Add/1  "kiteZcorrDepth"
  [estPosX] -> Sum4/1
  Gain34/1 -> Sum8/1
  Line Angle Sensor/3(thetaDot) -> thetaDot/1
  Line Angle Sensor/2(phiDot) -> phiDot/1
  [gndNodeTenVecs] -> Line Angle Sensor/5(thrLAStenVec)
  raftPsi/1 -> Line Angle Sensor/2(raftPsi)
  raftAcc/1 -> Line Angle Sensor/1(raftAcc)
  [flowSpd] -> Line Angle Sensor/6(flowSpd)
  Line Angle Sensor/4(theta) -> theta/1, [theta]
  raftPsiDot/1 -> Line Angle Sensor/3(raftPsiDot)
  raftPsiDDot/1 -> Line Angle Sensor/4(raftPsiDDot)
  [raftVel] -> Line Angle Sensor/7(raftVel)
  Line Angle Sensor/1(phi) -> phi/1, [phi]
  flowSpd/1 -> [flowSpd]
  Subsystem/2(bdy2Inert) -> [oCb_kite]
  kiteEulerAngles/1 -> Demux3/1
  Subsystem/1(inert2Bdy) -> Terminator11/1
  Demux3/2 -> Subsystem/2(pitch)
  Demux3/3 -> Subsystem/3(yaw)
  Demux3/1 -> Subsystem/1(roll)
  LASthetaMeas/1 -> Sum23/2
  Gain9/1 -> [kiteZcorrTheta]
  Mux2/1 -> Gain12/1
  Clock/1 -> Switch/2
  Gain19/1 -> Switch/3, Gain14/1
  Clock1/1 -> Switch1/2
  Switch1/1 -> Gain43/1
  Gain49/1 -> [kiteXcorrPhi]
  Cos/1 -> Divide2/2
  Tan/1 -> Divide2/1
  Divide2/1 -> Atan/1
  [theta] -> Tan/1
  [phi] -> Cos/1
  Gain47/1 -> Gain13/1, Switch2/3
  Clock2/1 -> Switch2/2
  Gain41/1 -> Switch1/1, Switch1/3
  Gain13/1 -> Switch2/1
  Gain14/1 -> Switch/1
  [kiteZcorrTens] -> Add1/3  "kiteZcorrTens"
  Sum31/1 -> [tensError], Switch3/1
  Clock3/1 -> Switch3/2
  Ground/1 -> Switch3/3
  Sum32/1 -> Gain18/1
  [kiteXcorrTens] -> Add14/4  "kiteXcorrTens"
  tensionMeas/1 -> Sum31/1
  Atan/1 -> Sum23/1
  Tether/5(kiteTensionVec) -> [kiteNodeTenVec]
  Product3/1 -> Demux1/1
  Normalize Vector/1 -> Product3/2
  [extPosVec] -> Normalize Vector/1
  Demux1/2 -> [kiteYcorrTens]
  [kiteYcorrTens] -> Add2/3  "kiteYcorrTens"
  Gain11/1 -> Goto23/1  "kiteZcorrTens"
  Gain10/1 -> Goto19/1  "kiteXcorrTens"
  Memory/1 -> Goto27/1
  Memory1/1 -> Goto24/1
  [thrYaccCorr] -> Tether/10(yCorr)
  [thrXaccCorr] -> Tether/9(xCorr)
  [thrZaccCorr] -> Tether/11(zCorr)

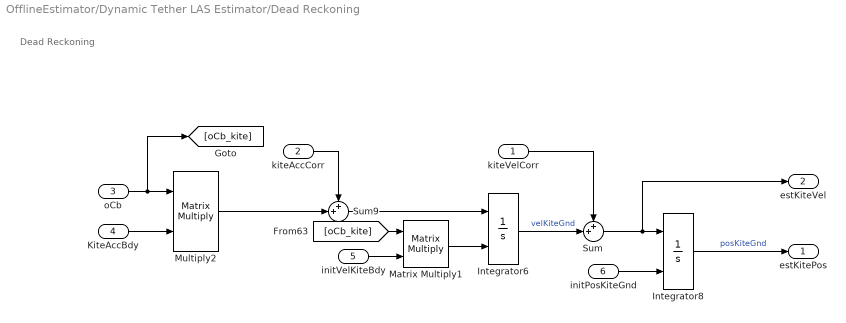
== system OfflineEstimator/Dynamic Tether LAS Estimator/Dead Reckoning ==
  note: Dead Reckoning
  kiteVelCorr : Inport
  kiteAccCorr : Inport  Port=2
  oCb : Inport  Port=3
  KiteAccBdy : Inport  Port=4
  initVelKiteBdy : Inport  Port=5
  initPosKiteGnd : Inport  Port=6
  Integrator6 : Integrator  InitialConditionSource=external
  Integrator8 : Integrator  InitialConditionSource=external
  Matrix Multiply1 : Product  Multiplication=Matrix(*)
  Multiply2 : Product  Multiplication=Matrix(*)
  Sum : Sum  Inputs=++|
  Sum9 : Sum  Inputs=++|
  estKitePos : Outport
  estKiteVel : Outport  Port=2
  wires:
  kiteAccCorr/1 -> Sum9/1
  initPosKiteGnd/1 -> Integrator8/2
  oCb/1 -> Multiply2/1, [oCb_kite]
  initVelKiteBdy/1 -> Matrix Multiply1/2
  kiteVelCorr/1 -> Sum/1
  KiteAccBdy/1 -> Multiply2/2
  Sum9/1 -> Integrator6/1
  Multiply2/1 -> Sum9/2
  Integrator6/1 -> Sum/2  "velKiteGnd"
  Integrator8/1 -> estKitePos/1  "posKiteGnd"
  [oCb_kite] -> Matrix Multiply1/1
  Matrix Multiply1/1 -> Integrator6/2
  Sum/1 -> Integrator8/1, estKiteVel/1

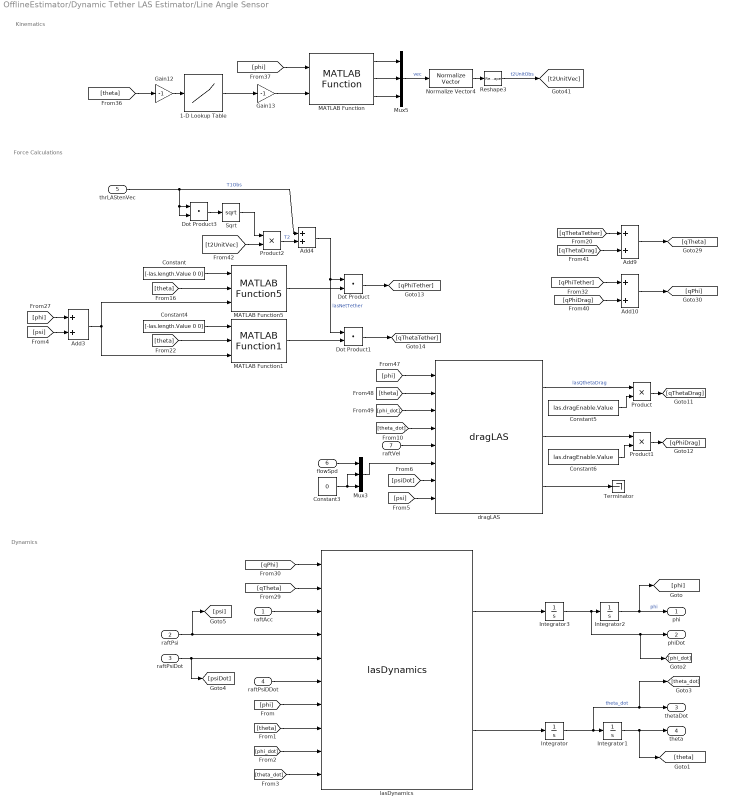
== system OfflineEstimator/Dynamic Tether LAS Estimator/Line Angle Sensor ==
  note: Dynamics
  note: Force Calculations
  note: Kinematics
  raftAcc : Inport
  raftPsi : Inport  Port=2
  raftPsiDot : Inport  Port=3
  raftPsiDDot : Inport  Port=4
  thrLAStenVec : Inport  Port=5
  flowSpd : Inport  Port=6
  raftVel : Inport  Port=7
  1-D Lookup Table : Lookup_n-D  NumberOfTableDimensions=1  BreakpointsForDimension1=las.thrAngLookup.Value(2,:)  Table=las.thrAngLookup.Value(1,:)  InternalRulePriority=Speed  RndMeth=Simplest  InputSameDT=on
  Add{3..4,9..10} (4 alike) : Sum
  Constant : Constant  Value=[-las.length.Value 0 0]
  Constant3 : Constant  Value=0
  Constant4 : Constant  Value=[-las.length.Value 0 0]
  Constant5 : Constant  Value=las.dragEnable.Value
  Constant6 : Constant  Value=las.dragEnable.Value
  Dot Product : DotProduct  InputSameDT=on  OutDataTypeStr=Inherit: Inherit via internal rule
  Dot Product1 : DotProduct  InputSameDT=on  OutDataTypeStr=Inherit: Inherit via internal rule
  Dot Product3 : DotProduct  InputSameDT=on  OutDataTypeStr=Inherit: Inherit via internal rule
  Gain12 : Gain  Gain=-1
  Gain13 : Gain  Gain=-1
  Integrator : Integrator  InitialCondition=obsLASthetadotInit
  Integrator1 : Integrator  InitialCondition=obsLASthetaInit
  Integrator2 : Integrator  InitialCondition=obsLASphiInit
  Integrator3 : Integrator  InitialCondition=obsLASphidotInit
  MATLAB Function : lineAngleSensor/lineAngleSensor/MATLAB Function  SystemSampleTime=-1  Latency=0  AutoFrameSizeCalculation=off
  MATLAB Function1 : lineAngleSensor/lineAngleSensor/MATLAB Function1  SystemSampleTime=-1  Latency=0  AutoFrameSizeCalculation=off
  MATLAB Function5 : lineAngleSensor/lineAngleSensor/MATLAB Function5  SystemSampleTime=-1  Latency=0  AutoFrameSizeCalculation=off
  Mux3 : Mux  Inputs=3
  Mux5 : Mux  Inputs=3
  Normalize Vector4 : vrlib/Utilities/Normalize Vector  maxzero=0
  Product : Product
  Product1 : Product
  Product2 : Product
  Reshape3 : Reshape  OutputDimensionality=Column vector (2-D)
  Sqrt : Sqrt  SaturateOnIntegerOverflow=on
  Terminator : Terminator
  dragLAS : lineAngleSensor/lineAngleSensor/dragLAS  rho=env.water.density.Value  C_D=las.CD.Value  L=las.length.Value  numDx=10  w=las.diameter.Value
  lasDynamics : lineAngleSensor/lineAngleSensor/lasDynamics  g=env.gravAccel.Value  mass_LAS=las.mass.Value  Fb_LAS=las.volume.Value*env.water.density.Value*env.gravAccel.Value  IxxLAS=las.Ixx.Value  IyyLAS=las.Iyy.Value  IzzLAS=las.Izz.Value  L_CB=las.L_CB.Value  L_CM=las.L_CM.Value
  phi : Outport
  phiDot : Outport  Port=2
  thetaDot : Outport  Port=3
  theta : Outport  Port=4
  wires:
  [psi] -> dragLAS/8
  [psi] -> Add3/2
  [psiDot] -> dragLAS/7
  raftAcc/1 -> lasDynamics/3
  lasDynamics/1 -> Integrator3/1
  [phi] -> dragLAS/1
  Dot Product1/1 -> [qThetaTether]
  raftPsi/1 -> lasDynamics/4, [psi]
  [theta] -> dragLAS/2
  dragLAS/1 -> Product/1  "lasQthetaDrag"
  [phi] -> lasDynamics/7
  [theta] -> MATLAB Function5/2
  lasDynamics/2 -> Integrator/1
  [qPhi] -> lasDynamics/1
  Mux3/1 -> dragLAS/6
  raftPsiDot/1 -> lasDynamics/5, [psiDot]
  MATLAB Function5/1 -> Dot Product/2
  Reshape3/1 -> [t2UnitVec]  "t2UnitObs"
  Constant6/1 -> Product1/2
  [qThetaTether] -> Add9/1
  MATLAB Function1/1 -> Dot Product1/2
  Normalize Vector4/1 -> Reshape3/1
  [qThetaDrag] -> Add9/2
  Add9/1 -> [qTheta]
  [qTheta] -> lasDynamics/2
  [theta] -> lasDynamics/8
  raftVel/1 -> dragLAS/5
  Add10/1 -> [qPhi]
  Dot Product/1 -> [qPhiTether]
  MATLAB Function/3 -> Mux5/3
  Product/1 -> [qThetaDrag]
  thrLAStenVec/1 -> Dot Product3/1, Dot Product3/2, Add4/1  "T1Obs"
  Gain12/1 -> 1-D Lookup Table/1
  [phi_dot] -> lasDynamics/9
  Gain13/1 -> MATLAB Function/2
  [phi] -> MATLAB Function/1
  [theta] -> Gain12/1
  [phi] -> Add3/1
  Constant3/1 -> Mux3/3, Mux3/2
  Constant/1 -> MATLAB Function5/1
  raftPsiDDot/1 -> lasDynamics/6
  MATLAB Function/2 -> Mux5/2
  Constant5/1 -> Product/2
  [qPhiTether] -> Add10/1
  [theta_dot] -> dragLAS/4
  Dot Product3/1 -> Sqrt/1
  Add4/1 -> Dot Product/1, Dot Product1/1  "lasNetTether"
  Add3/1 -> MATLAB Function1/3, MATLAB Function5/3
  dragLAS/2 -> Product1/1
  Integrator1/1 -> theta/1, [theta]
  Product1/1 -> [qPhiDrag]
  1-D Lookup Table/1 -> Gain13/1
  dragLAS/3 -> Terminator/1
  [t2UnitVec] -> Product2/2
  Sqrt/1 -> Product2/1
  Integrator/1 -> Integrator1/1, thetaDot/1, [theta_dot]  "theta_dot"
  Integrator2/1 -> phi/1, [phi]  "phi"
  Mux5/1 -> Normalize Vector4/1  "vec"
  [theta_dot] -> lasDynamics/10
  Product2/1 -> Add4/2  "T2"
  flowSpd/1 -> Mux3/1
  Constant4/1 -> MATLAB Function1/1
  [qPhiDrag] -> Add10/2
  MATLAB Function/1 -> Mux5/1
  Integrator3/1 -> phiDot/1, [phi_dot], Integrator2/1
  [theta] -> MATLAB Function1/2
  [phi_dot] -> dragLAS/3

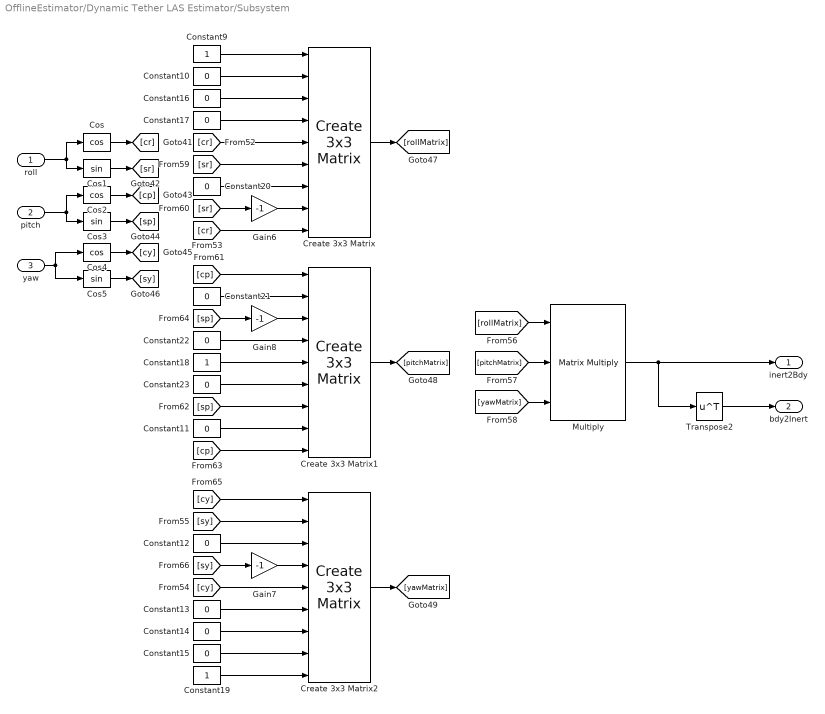
== system OfflineEstimator/Dynamic Tether LAS Estimator/Subsystem ==
  roll : Inport
  pitch : Inport  Port=2
  yaw : Inport  Port=3
  Constant{10..17,20..23} (12 alike) : Constant  Value=0
  Constant18 : Constant
  Constant19 : Constant
  Constant9 : Constant
  Cos : Trigonometry  Operator=cos
  Cos1 : Trigonometry
  Cos2 : Trigonometry  Operator=cos
  Cos3 : Trigonometry
  Cos4 : Trigonometry  Operator=cos
  Cos5 : Trigonometry
  Create 3x3 Matrix : sharedutil/Create 3x3 Matrix  aMode=aMode
  Create 3x3 Matrix1 : sharedutil/Create 3x3 Matrix  aMode=aMode
  Create 3x3 Matrix2 : sharedutil/Create 3x3 Matrix  aMode=aMode
  Gain6 : Gain  Gain=-1
  Gain7 : Gain  Gain=-1
  Gain8 : Gain  Gain=-1
  Multiply : Product  Inputs=3  Multiplication=Matrix(*)
  Transpose2 : Math  Operator=transpose  SignedPower=on  SaturateOnIntegerOverflow=on
  inert2Bdy : Outport  VectorParamsAs1DForOutWhenUnconnected=off
  bdy2Inert : Outport  Port=2  VectorParamsAs1DForOutWhenUnconnected=off
  wires:
  [cp] -> Create 3x3 Matrix1/1
  Cos/1 -> [cr]
  [cr] -> Create 3x3 Matrix/5
  Constant23/1 -> Create 3x3 Matrix1/6
  Constant9/1 -> Create 3x3 Matrix/1
  Cos3/1 -> [sp]
  [pitchMatrix] -> Multiply/2
  pitch/1 -> Cos3/1, Cos2/1
  [yawMatrix] -> Multiply/3
  [sy] -> Create 3x3 Matrix2/2
  Cos1/1 -> [sr]
  Constant20/1 -> Create 3x3 Matrix/7
  Gain8/1 -> Create 3x3 Matrix1/3
  Constant18/1 -> Create 3x3 Matrix1/5
  [sp] -> Create 3x3 Matrix1/7
  Create 3x3 Matrix1/1 -> [pitchMatrix]
  Constant19/1 -> Create 3x3 Matrix2/9
  Constant14/1 -> Create 3x3 Matrix2/7
  Constant11/1 -> Create 3x3 Matrix1/8
  Gain6/1 -> Create 3x3 Matrix/8
  Multiply/1 -> Transpose2/1, inert2Bdy/1
  roll/1 -> Cos/1, Cos1/1
  [cp] -> Create 3x3 Matrix1/9
  Constant15/1 -> Create 3x3 Matrix2/8
  Constant21/1 -> Create 3x3 Matrix1/2
  Constant13/1 -> Create 3x3 Matrix2/6
  Gain7/1 -> Create 3x3 Matrix2/4
  Constant16/1 -> Create 3x3 Matrix/3
  Constant22/1 -> Create 3x3 Matrix1/4
  Constant10/1 -> Create 3x3 Matrix/2
  [sr] -> Gain6/1
  [cy] -> Create 3x3 Matrix2/1
  Create 3x3 Matrix/1 -> [rollMatrix]
  Constant17/1 -> Create 3x3 Matrix/4
  Cos4/1 -> [cy]
  [sp] -> Gain8/1
  yaw/1 -> Cos4/1, Cos5/1
  [cr] -> Create 3x3 Matrix/9
  Create 3x3 Matrix2/1 -> [yawMatrix]
  [sy] -> Gain7/1
  [sr] -> Create 3x3 Matrix/6
  Cos2/1 -> [cp]
  [rollMatrix] -> Multiply/1
  [cy] -> Create 3x3 Matrix2/5
  Constant12/1 -> Create 3x3 Matrix2/3
  Transpose2/1 -> bdy2Inert/1
  Cos5/1 -> [sy]

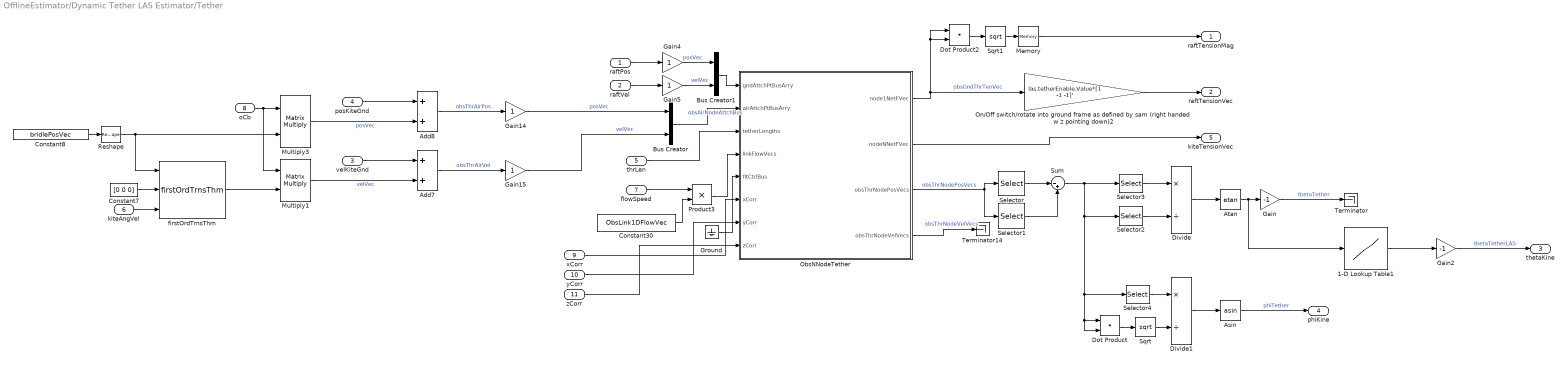
== system OfflineEstimator/Dynamic Tether LAS Estimator/Tether ==
  raftPos : Inport
  raftVel : Inport  Port=2
  velKiteGnd : Inport  Port=3
  posKiteGnd : Inport  Port=4
  thrLen : Inport  Port=5
  kiteAngVel : Inport  Port=6
  flowSpeed : Inport  Port=7
  oCb : Inport  Port=8
  xCorr : Inport  Port=9
  yCorr : Inport  Port=10
  zCorr : Inport  Port=11
  1-D Lookup Table1 : Lookup_n-D  NumberOfTableDimensions=1  BreakpointsForDimension1=las.thrAngLookup.Value(1,:)  Table=las.thrAngLookup.Value(2,:)  InternalRulePriority=Speed  RndMeth=Simplest  InputSameDT=on
  Add7 : Sum
  Add8 : Sum
  Asin : Trigonometry  Operator=asin
  Atan : Trigonometry  Operator=atan
  Bus Creator : BusCreator  Inputs=2  OutDataTypeStr=Bus: thrAttachPtKinematicsBus  NonVirtualBus=on
  Bus Creator1 : BusCreator  Inputs=2  OutDataTypeStr=Bus: thrAttachPtKinematicsBus  NonVirtualBus=on
  Constant30 : Constant  Value=ObsLink1DFlowVec
  Constant7 : Constant  Value=[0 0 0]
  Constant8 : Constant  Value=bridlePosVec
  Divide : Product  Inputs=*/
  Divide1 : Product  Inputs=*/
  Dot Product : DotProduct  InputSameDT=on  OutDataTypeStr=Inherit: Inherit via internal rule
  Dot Product2 : DotProduct  InputSameDT=on  OutDataTypeStr=Inherit: Inherit via internal rule
  Gain : Gain  Gain=-1
  Gain{4..5,14..15} (4 alike) : Gain
  Gain2 : Gain  Gain=-1
  Ground : Ground
  Memory : Memory
  Multiply1 : Product  Multiplication=Matrix(*)
  Multiply3 : Product  Multiplication=Matrix(*)
  ObsNNodeTether : Subsystem  Variant=on  VariantControl=NNodeTether
  On/Off switch/rotate into ground frame as defined by sam (right handed w z pointing down)2 : Gain  Gain=las.tetherEnable.Value*[1 -1 -1]'
  Product3 : Product
  Reshape : Reshape  OutputDimensionality=Column vector (2-D)
  Selector : Selector  NumberOfDimensions=2  InputPortWidth=3  IndexOptions=Index vector (dialog),Index vector (dialog)  Indices=[1 2 3],1  OutputSizes=1,1
  Selector1 : Selector  NumberOfDimensions=2  InputPortWidth=3  IndexOptions=Index vector (dialog),Index vector (dialog)  Indices=[1 2 3],2  OutputSizes=1,1
  Selector2 : Selector  InputPortWidth=3  IndexOptions=Index vector (dialog)  Indices=[1]  OutputSizes=1
  Selector3 : Selector  InputPortWidth=3  IndexOptions=Index vector (dialog)  Indices=[3]  OutputSizes=1
  Selector4 : Selector  InputPortWidth=3  IndexOptions=Index vector (dialog)  Indices=[2]  OutputSizes=1
  Sqrt : Sqrt  SaturateOnIntegerOverflow=on
  Sqrt1 : Sqrt  SaturateOnIntegerOverflow=on
  Sum : Sum  Inputs=|-+
  Terminator : Terminator
  Terminator14 : Terminator
  firstOrdTrnsThm : firstOrdTrnsThm_ul/firstOrdTrnsThm  SystemSampleTime=-1  Latency=0  AutoFrameSizeCalculation=off
  raftTensionMag : Outport
  raftTensionVec : Outport  Port=2
  thetaKine : Outport  Port=3
  phiKine : Outport  Port=4
  kiteTensionVec : Outport  Port=5
  wires:
  Sum/1 -> Selector3/1, Dot Product/2, Dot Product/1, Selector4/1, Selector2/1
  Asin/1 -> phiKine/1  "phiTether"
  Dot Product/1 -> Sqrt/1
  Sqrt/1 -> Divide1/2
  Selector4/1 -> Divide1/1
  Divide1/1 -> Asin/1
  Atan/1 -> Gain/1, 1-D Lookup Table1/1
  1-D Lookup Table1/1 -> Gain2/1
  Gain2/1 -> thetaKine/1  "thetaTetherLAS"
  Gain/1 -> Terminator/1  "thetaTether"
  Divide/1 -> Atan/1
  Selector2/1 -> Divide/2
  Selector3/1 -> Divide/1
  Selector1/1 -> Sum/2
  Selector/1 -> Sum/1
  Product3/1 -> ObsNNodeTether/4(linkFlowVecs)
  Constant30/1 -> Product3/2
  Gain5/1 -> Bus Creator1/2  "velVec"
  ObsNNodeTether/3(obsThrNodePosVecs) -> Selector/1, Selector1/1  "obsThrNodePosVecs"
  flowSpeed/1 -> Product3/1
  Bus Creator/1 -> ObsNNodeTether/2(airAttchPtBusArry)  "obsAirNodeAttchBus"
  Memory/1 -> raftTensionMag/1
  Gain14/1 -> Bus Creator/1  "posVec"
  Ground/1 -> ObsNNodeTether/5(fltCtrlBus)
  oCb/1 -> Multiply3/1, Multiply1/1
  ObsNNodeTether/2(nodeNNetFVec) -> kiteTensionVec/1
  posKiteGnd/1 -> Add8/1
  Dot Product2/1 -> Sqrt1/1
  kiteAngVel/1 -> firstOrdTrnsThm/3
  Bus Creator1/1 -> ObsNNodeTether/1(gndAttchPtBusArry)
  thrLen/1 -> ObsNNodeTether/3(tetherLengths)
  ObsNNodeTether/1(node1NetFVec) -> Dot Product2/2, Dot Product2/1, On/Off switch/rotate into ground frame as defined by sam (right handed w z pointing down)2/1  "obsGndThrTenVec"
  velKiteGnd/1 -> Add7/1
  Reshape/1 -> Multiply3/2, firstOrdTrnsThm/1
  Gain15/1 -> Bus Creator/2  "velVec"
  firstOrdTrnsThm/1 -> Multiply1/2
  Multiply1/1 -> Add7/2  "velVec"
  Constant7/1 -> firstOrdTrnsThm/2
  Multiply3/1 -> Add8/2  "posVec"
  Add7/1 -> Gain15/1  "obsThrAirVel"
  raftVel/1 -> Gain5/1
  Add8/1 -> Gain14/1  "obsThrAirPos"
  ObsNNodeTether/4(obsThrNodeVelVecs) -> Terminator14/1  "obsThrNodeVelVecs"
  On/Off switch/rotate into ground frame as defined by sam (right handed w z pointing down)2/1 -> raftTensionVec/1
  Sqrt1/1 -> Memory/1
  Gain4/1 -> Bus Creator1/1  "posVec"
  raftPos/1 -> Gain4/1
  Constant8/1 -> Reshape/1
  xCorr/1 -> ObsNNodeTether/6(xCorr)
  yCorr/1 -> ObsNNodeTether/7(yCorr)
  zCorr/1 -> ObsNNodeTether/8(zCorr)

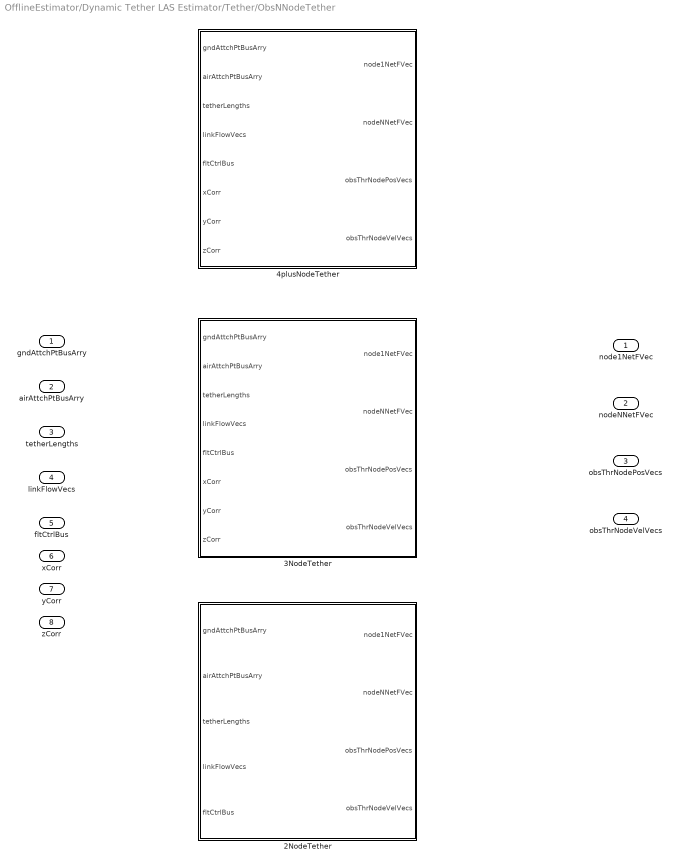
== system OfflineEstimator/Dynamic Tether LAS Estimator/Tether/ObsNNodeTether ==
  gndAttchPtBusArry : Inport
  airAttchPtBusArry : Inport  Port=2
  tetherLengths : Inport  Port=3
  linkFlowVecs : Inport  Port=4
  fltCtrlBus : Inport  Port=5
  xCorr : Inport  Port=6
  yCorr : Inport  Port=7
  zCorr : Inport  Port=8
  2NodeTether : Subsystem  VariantControl=strcmpi(OBSTETHER,'2NodeTether')  mask{thr=Obsthr.struct('OCT.tether'), flowDensity=env.water.density.Value, gravity=env.gravAccel.Value, numNodes=Obsthr.numNodes.Value}
      mask prompts: thr "Tether Structure"; flowDensity "Fluid Density"; gravity "Gravitational Acceleration"; numNodes "Number of Nodes"
  3NodeTether : Subsystem  VariantControl=strcmpi(OBSTETHER,'3NodeTether')  mask{thr=Obsthr.struct('OCT.tether'), flowDensity=env.water.density.Value, gravity=env.gravAccel.Value, numNodes=Obsthr.numNodes.Value}
      mask prompts: thr "Tether Structure"; flowDensity "Fluid Density"; gravity "Gravitational Acceleration"; numNodes "Number of Nodes"
  4plusNodeTether : Subsystem  AncestorBlock=NNodeTether_cl/NNodeTether  VariantControl=strcmpi(OBSTETHER,'4plusNodeTether')  mask{thr=Obsthr.struct('OCT.tether'), flowDensity=env.water.density.Value, gravity=env.gravAccel.Value, numNodes=Obsthr.numNodes.Value}
      mask prompts: thr "Tether Structure"; flowDensity "Fluid Density"; gravity "Gravitational Acceleration"; numNodes "Number of Nodes"
  node1NetFVec : Outport
  nodeNNetFVec : Outport  Port=2
  obsThrNodePosVecs : Outport  Port=3
  obsThrNodeVelVecs : Outport  Port=4
